simulink model "bicycle_model"  (R2013b)
settings: Solver=ode3  StartTime=0.0  StopTime=6.0  FixedStep=0.01  RelTol=1e-3
InitFcn:
  | mass = 9;
  | wheelbase = 0.5;
  | cgDistFromRear = 0.25;
  | Cf = -(cgDistFromRear/wheelbase*100)*mass*9.81*0.17;
  | Cr = -(100-(cgDistFromRear/wheelbase*100))*mass*9.81*0.17;
  | v = 20;
  | J = 0.5;
  | 
  | 
  | a = wheelbase - cgDistFromRear;
  | b = cgDistFromRear;
settings Model: Creator=Lasse  LastModifiedBy=kortetl1

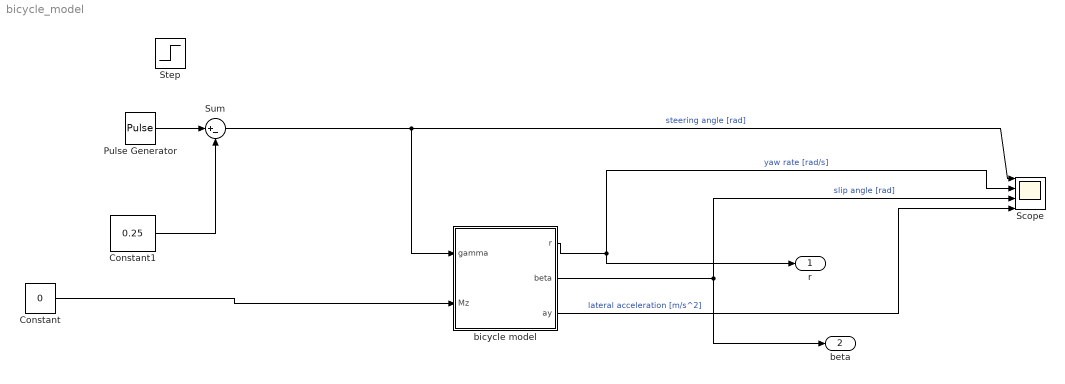
== system bicycle_model ==
  Constant : Constant  Value=0
  Constant1 : Constant  Value=0.25
  Pulse Generator : DiscretePulseGenerator  PulseType=Time based  Amplitude=0.5  PulseWidth=50
  Scope : Scope  NumInputPorts=4
      settings: YMin=0~-5~-5~-5  YMax=0.1~5~5~5
  Step : Step  After=0.0125  SampleTime=0
  Sum : Sum  Inputs=|+-
  bicycle model : Subsystem
  r : Outport
  beta : Outport  Port=2
  wires:
  Pulse Generator/1 -> Sum/1
  Constant1/1 -> Sum/2
  Sum/1 -> bicycle model/1(gamma), Scope/1  "steering angle [rad]"
  bicycle model/1(r) -> r/1, Scope/2  "yaw rate [rad/s]"
  bicycle model/2(beta) -> beta/1, Scope/3  "slip angle [rad]"
  Constant/1 -> bicycle model/2(Mz)
  bicycle model/3(ay) -> Scope/4  "lateral acceleration [m/s^2]"

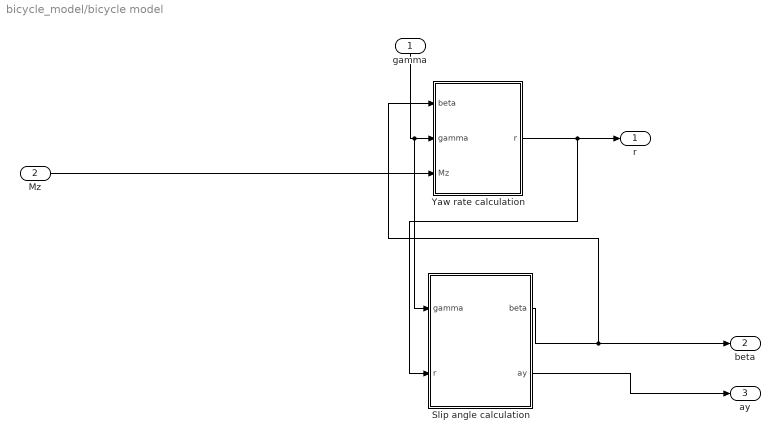
== system bicycle_model/bicycle model ==
  gamma : Inport
  Mz : Inport  Port=2
  Slip angle calculation : Subsystem
  Yaw rate calculation : Subsystem
  r : Outport
  beta : Outport  Port=2
  ay : Outport  Port=3
  wires:
  Yaw rate calculation/1(r) -> r/1, Slip angle calculation/2(r)
  Slip angle calculation/1(beta) -> beta/1, Yaw rate calculation/1(beta)
  Mz/1 -> Yaw rate calculation/3(Mz)
  gamma/1 -> Slip angle calculation/1(gamma), Yaw rate calculation/2(gamma)
  Slip angle calculation/2(ay) -> ay/1

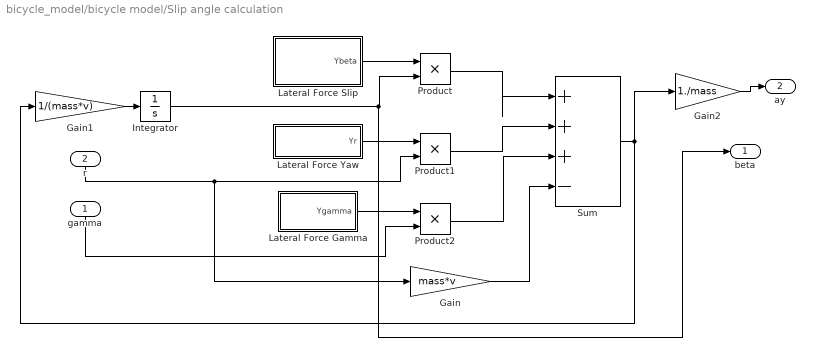
== system bicycle_model/bicycle model/Slip angle calculation ==
  gamma : Inport
  r : Inport  Port=2
  Gain : Gain  Gain=mass*v
  Gain1 : Gain  Gain=1/(mass*v)
  Gain2 : Gain  Gain=1./mass
  Integrator : Integrator
  Lateral Force Gamma : Subsystem
  "Lateral Force Slip " : Subsystem
  Lateral Force Yaw : Subsystem
  Product : Product
  Product1 : Product
  Product2 : Product
  Sum : Sum  Inputs=|+++-
  beta : Outport
  ay : Outport  Port=2
  wires:
  gamma/1 -> Product2/2
  r/1 -> Product1/2, Gain/1
  "Lateral Force Slip "/1(Ybeta) -> Product/1
  Lateral Force Yaw/1(Yr) -> Product1/1
  Sum/1 -> Gain1/1, Gain2/1
  Product/1 -> Sum/1
  Lateral Force Gamma/1(Ygamma) -> Product2/1
  Gain1/1 -> Integrator/1
  Product2/1 -> Sum/3
  Integrator/1 -> beta/1, Product/2
  Product1/1 -> Sum/2
  Gain/1 -> Sum/4
  Gain2/1 -> ay/1

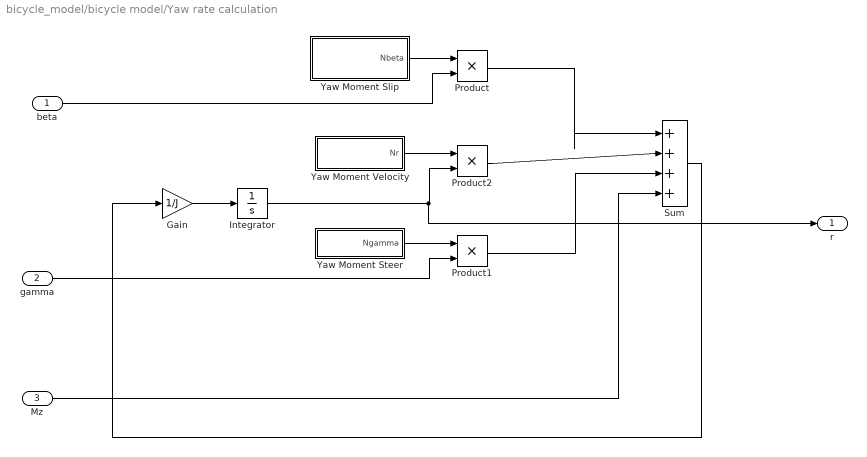
== system bicycle_model/bicycle model/Yaw rate calculation ==
  beta : Inport
  gamma : Inport  Port=2
  Mz : Inport  Port=3
  Gain : Gain  Gain=1/J
  Integrator : Integrator
  Product : Product
  Product1 : Product
  Product2 : Product
  Sum : Sum  Inputs=|++++
  Yaw Moment Slip : Subsystem
  Yaw Moment Steer : Subsystem
  Yaw Moment Velocity : Subsystem
  r : Outport
  wires:
  Yaw Moment Slip/1(Nbeta) -> Product/1
  Product2/1 -> Sum/2
  Yaw Moment Steer/1(Ngamma) -> Product1/1
  Product1/1 -> Sum/3
  beta/1 -> Product/2
  Yaw Moment Velocity/1(Nr) -> Product2/1
  Integrator/1 -> r/1, Product2/2
  Product/1 -> Sum/1
  Mz/1 -> Sum/4
  gamma/1 -> Product1/2
  Sum/1 -> Gain/1
  Gain/1 -> Integrator/1

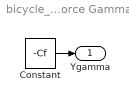
== system bicycle_model/bicycle model/Slip angle calculation/Lateral Force Gamma ==
  Constant : Constant  Value=-Cf
  Ygamma : Outport
  wires:
  Constant/1 -> Ygamma/1

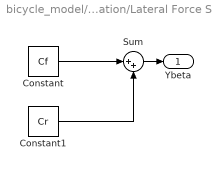
== system bicycle_model/bicycle model/Slip angle calculation/Lateral Force Slip  ==
  Constant : Constant  Value=Cf
  Constant1 : Constant  Value=Cr
  Sum : Sum  Inputs=|++
  Ybeta : Outport
  wires:
  Sum/1 -> Ybeta/1
  Constant1/1 -> Sum/2
  Constant/1 -> Sum/1

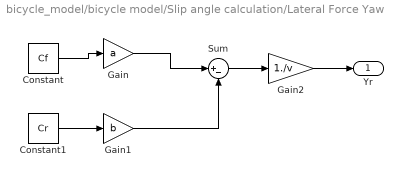
== system bicycle_model/bicycle model/Slip angle calculation/Lateral Force Yaw ==
  Constant : Constant  Value=Cf
  Constant1 : Constant  Value=Cr
  Gain : Gain  Gain=a
  Gain1 : Gain  Gain=b
  Gain2 : Gain  Gain=1./v
  Sum : Sum  Inputs=|+-
  Yr : Outport
  wires:
  Sum/1 -> Gain2/1
  Gain/1 -> Sum/1
  Constant/1 -> Gain/1
  Constant1/1 -> Gain1/1
  Gain1/1 -> Sum/2
  Gain2/1 -> Yr/1

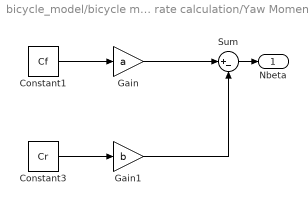
== system bicycle_model/bicycle model/Yaw rate calculation/Yaw Moment Slip ==
  Constant1 : Constant  Value=Cf
  Constant3 : Constant  Value=Cr
  Gain : Gain  Gain=a
  Gain1 : Gain  Gain=b
  Sum : Sum  Inputs=|+-
  Nbeta : Outport
  wires:
  Sum/1 -> Nbeta/1
  Constant3/1 -> Gain1/1
  Constant1/1 -> Gain/1
  Gain1/1 -> Sum/2
  Gain/1 -> Sum/1

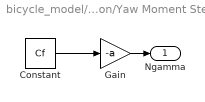
== system bicycle_model/bicycle model/Yaw rate calculation/Yaw Moment Steer ==
  Constant : Constant  Value=Cf
  Gain : Gain  Gain=-a
  Ngamma : Outport
  wires:
  Gain/1 -> Ngamma/1
  Constant/1 -> Gain/1

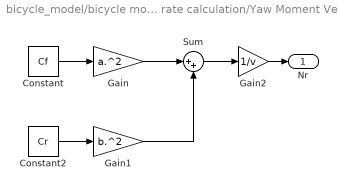
== system bicycle_model/bicycle model/Yaw rate calculation/Yaw Moment Velocity ==
  Constant : Constant  Value=Cf
  Constant2 : Constant  Value=Cr
  Gain : Gain  Gain=a.^2
  Gain1 : Gain  Gain=b.^2
  Gain2 : Gain  Gain=1/v
  Sum : Sum  Inputs=|++
  Nr : Outport
  wires:
  Gain2/1 -> Nr/1
  Gain/1 -> Sum/1
  Constant/1 -> Gain/1
  Gain1/1 -> Sum/2
  Sum/1 -> Gain2/1
  Constant2/1 -> Gain1/1
